simulink model "new_dynamics_sim"  (R2019b)
settings: Solver=VariableStepAuto  StartTime=0.0  StopTime=100  RelTol=1e-3
values from neighbouring files (symbols this model uses):
  A = [0 0       0        1 ... (first row only)    [fbexample.m]    (also in new_dynamics.m = [A_longitude_hi(2,2), A_longitude_hi(2,4), A_longitude_hi(2,; setup_sim.m = A_hi; x29soln.m = [  -0.1645   0.0603 -0.9982 0.0442)
  B = [       0 ... (first row only)    [fbexample.m]    (also in new_dynamics.m = [A_longitude_hi(2, end), A_longitude_hi(4, end), A_longitude; setup_sim.m = B_hi; x29soln.m = [-0.0006  0.0007)
  C = eye(4)    [fbexample.m]    (also in new_dynamics.m = eye(3); second_week.m = pid(-2.29,-1.15); setup_sim.m = eye(18); x29soln.m)
  D = 0    [fbexample.m]    (also in new_dynamics.m = zeros(3,1); setup_sim.m = zeros(18,4); x29soln.m = zeros(4,2))
undefined symbols (not defined in the file or in its folder): K_pr
libraries: simulink_extras x2
settings Model: Creator=wagneda1  LastModifiedBy=asmialek
settings DataIOCC: ReturnWorkspaceOutputs=off
settings DebuggingCC: ArithmeticOperatorsInVariantConditions=warning
settings SFSimCC: SimUseLocalCustomCode=off  CustomCodeUndefinedFunction=UseInterfaceOnly
settings RTWCC: RTWUseLocalCustomCode=off
settings CodeAppCC: StateflowObjectComments=on

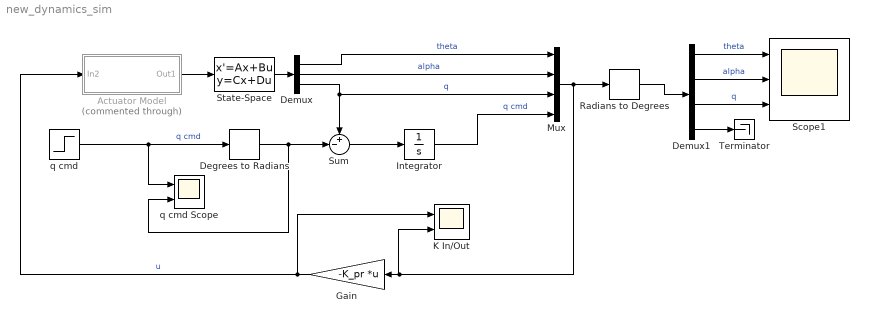
== system new_dynamics_sim ==
  Actuator Model : Subsystem  Commented=through
  Degrees to Radians : simulink_extras/Transformations/Degrees to Radians
  Demux : Demux  Outputs=3
  Demux1 : Demux
  Gain : Gain  Gain=-K_pr  Multiplication=Matrix(K*u)
  Integrator : Integrator
  K In/Out : Scope  NumInputPorts=2
  Mux : Mux
  Radians to Degrees : simulink_extras/Transformations/Radians to Degrees
  Scope1 : Scope  NumInputPorts=3
  State-Space : StateSpace  A=A  B=B  C=C  D=D  InitialCondition=[ 0 deg2rad(5) 0 ]
  Sum : Sum  Inputs=+-|
  Terminator : Terminator
  q cmd : Step  Time=20  After=20  SampleTime=0  ZeroCross=off
  q cmd Scope : Scope  NumInputPorts=2
  wires:
  State-Space/1 -> Demux/1
  Demux/1 -> Mux/1  "theta"
  Demux/2 -> Mux/2  "alpha"
  Demux/3 -> Sum/1, Mux/3  "q"
  Sum/1 -> Integrator/1
  Gain/1 -> Actuator Model/1(In2), K In/Out/1  "u"
  q cmd/1 -> q cmd Scope/1, Degrees to Radians/1  "q cmd"
  Radians to Degrees/1 -> Demux1/1
  Degrees to Radians/1 -> q cmd Scope/2, Sum/2
  Actuator Model/1(Out1) -> State-Space/1
  Demux1/1 -> Scope1/1  "theta"
  Demux1/2 -> Scope1/2  "alpha"
  Demux1/3 -> Scope1/3  "q"
  Integrator/1 -> Mux/4  "q cmd"
  Mux/1 -> Radians to Degrees/1, K In/Out/2, Gain/1
  Demux1/4 -> Terminator/1

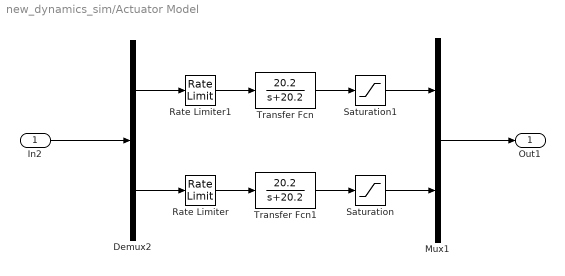
== system new_dynamics_sim/Actuator Model ==
  In2 : Inport
  Demux2 : Demux  Outputs=2
  Mux1 : Mux  Inputs=2
  Rate Limiter : RateLimiter  RisingSlewLimit=60  FallingSlewLimit=-60  SampleTimeMode=inherited
  Rate Limiter1 : RateLimiter  RisingSlewLimit=60  FallingSlewLimit=-60  SampleTimeMode=inherited
  Saturation : Saturate  UpperLimit=25  LowerLimit=-25
  Saturation1 : Saturate  UpperLimit=25  LowerLimit=-25
  Transfer Fcn : TransferFcn  Numerator=[20.2]  Denominator=[1 20.2]
  Transfer Fcn1 : TransferFcn  Numerator=[20.2]  Denominator=[1 20.2]
  Out1 : Outport
  wires:
  Mux1/1 -> Out1/1
  In2/1 -> Demux2/1
  Transfer Fcn1/1 -> Saturation/1
  Saturation/1 -> Mux1/2
  Transfer Fcn/1 -> Saturation1/1
  Saturation1/1 -> Mux1/1
  Rate Limiter/1 -> Transfer Fcn1/1
  Demux2/2 -> Rate Limiter/1
  Rate Limiter1/1 -> Transfer Fcn/1
  Demux2/1 -> Rate Limiter1/1
